simulink model "dlbsTestHarnessSplit3"  (R2025b)
settings: Solver=VariableStepAuto  StartTime=0.0  StopTime=10.0  RelTol=1e-3
undefined symbols (not defined in the file or in its folder): dY1, dY2, dY3, X
libraries: dlbsBlockInsertGradientGF x3, dlbsBlockExtractGradientGF x1, dlbsBlockSplit x1
settings Model: Creator=lt6037  LastModifiedBy=lt6037

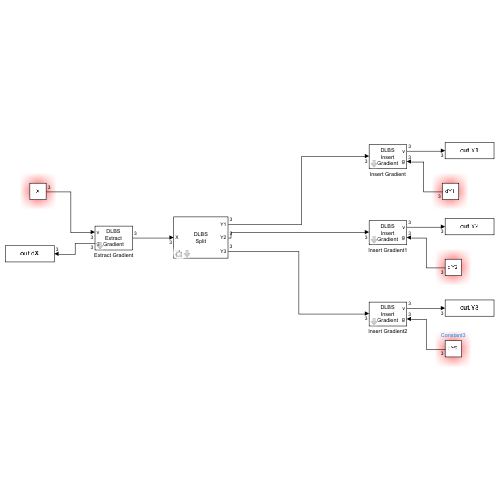
[thumbnail: Simulink's stored preview of the top-level diagram]
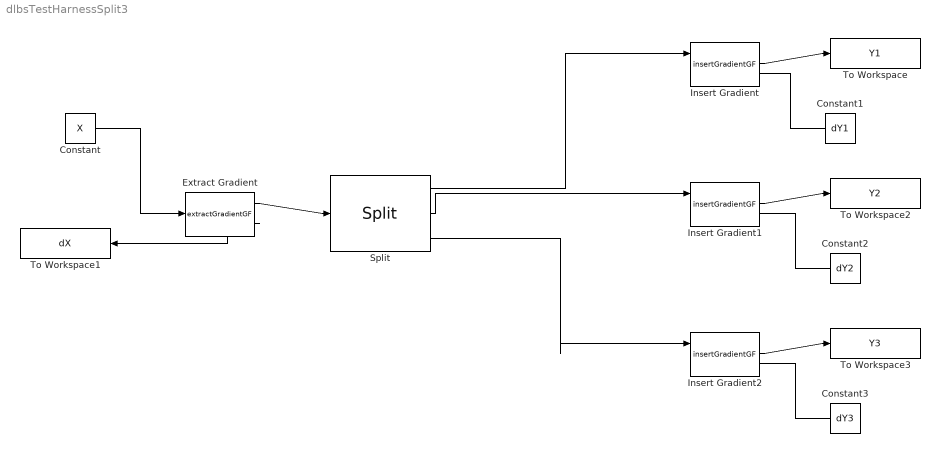
== system dlbsTestHarnessSplit3 ==
  Constant : Constant  Value=X  VectorParams1D=off
  Constant1 : Constant  Value=dY1  VectorParams1D=off
  Constant2 : Constant  Value=dY2  VectorParams1D=off
  Constant3 : Constant  Value=dY3  VectorParams1D=off
  Extract Gradient : dlbsBlockExtractGradientGF/extractGradientGF
  Insert Gradient : dlbsBlockInsertGradientGF/insertGradientGF
  Insert Gradient1 : dlbsBlockInsertGradientGF/insertGradientGF
  Insert Gradient2 : dlbsBlockInsertGradientGF/insertGradientGF
  Split : dlbsBlockSplit/Split  n_out=3  g1=on  g2=on  g3=on  g4=on
  To Workspace : ToWorkspace  VariableName=Y1  SaveFormat=Timeseries  SampleTime=-1
      settings: MaxDataPoints=1
  To Workspace1 : ToWorkspace  VariableName=dX  SaveFormat=Timeseries  SampleTime=-1
      settings: MaxDataPoints=1
  To Workspace2 : ToWorkspace  VariableName=Y2  SaveFormat=Timeseries  SampleTime=-1
      settings: MaxDataPoints=1
  To Workspace3 : ToWorkspace  VariableName=Y3  SaveFormat=Timeseries  SampleTime=-1
      settings: MaxDataPoints=1
  wires:
  Extract Gradient/2 -> To Workspace1/1
  Constant1/1 -> Insert Gradient/2
  Insert Gradient/1 -> To Workspace/1
  Split/1 -> Insert Gradient/1
  Constant/1 -> Extract Gradient/1
  Extract Gradient/1 -> Split/1
  Insert Gradient1/1 -> To Workspace2/1
  Constant2/1 -> Insert Gradient1/2
  Insert Gradient2/1 -> To Workspace3/1
  Constant3/1 -> Insert Gradient2/2
  Split/2 -> Insert Gradient1/1
  Split/3 -> Insert Gradient2/1
